simulink model "PassStBkReclnCtrl"  (R2018b)
settings: Solver=FixedStepDiscrete  StartTime=0.0  StopTime=10.0  RelTol=1e-3
undefined symbols (not defined in the file or in its folder): KeSMSuMdMotFinshdTm_Val, KeSMSuMdRetryTm1_Val, KeSMSuModeReqDurgTm_Val
libraries: StCtrlLibBkRecln x1
settings Model: Creator=sn2xws  LastModifiedBy=sn2xws
settings Model: ModifiedHistory=|
  | 2024.6.26 V3.0.0 557模式流程
  | 2024.8.23 V3.0.1更新Entrig接口
  | 2024.11.6 V3.0.2 模式流程V2.6 Md30 增加靠背目标位置1
settings DataIOCC: SaveFormat=StructureWithTime
settings OptimizationCC: DefaultParameterBehavior=Inlined  EnhancedBackFolding=on  PassReuseOutputArgsAs=Individual arguments  ZeroExternalMemoryAtStartup=off  ZeroInternalMemoryAtStartup=off  OptimizeBlockOrder=speed  DifferentSizesBufferReuse=on  OptimizationCustomize=off
settings DebuggingCC: ParameterTunabilityLossMsg=error
settings SFSimCC: MATLABDynamicMemAlloc=off
settings RTWCC: SystemTargetFile=autosar.tlc  GenCodeOnly=on  TemplateMakefile=ert_default_tmf  Description=AUTOSAR  GenerateReport=on  IncludeHyperlinkInReport=on  LaunchReport=on  GenerateTraceInfo=on  GenerateTraceReport=on  GenerateTraceReportSl=on  GenerateTraceReportSf=on  GenerateTraceReportEml=on
settings CodeAppCC: ForceParamTrailComments=on  IgnoreCustomStorageClasses=off  OperatorAnnotations=on  SimulinkDataObjDesc=on  SFDataObjDesc=on  InsertBlockDesc=on
settings STFCustomTargetCC: TargetLangStandard=C99 (ISO)  MultiwordLength=256  ParMdlRefBuildCompliant=on  CompOptLevelCompliant=on  IncludeMdlTerminateFcn=off  CombineOutputUpdateFcns=on  SuppressErrorStatus=on  ERTCustomFileBanners=on  SupportNonFinite=off  SupportComplex=off  SupportContinuousTime=off  SupportNonInlinedSFcns=off  RemoveResetFunc=on  MATLABClassNameForMDSCustomization=Simulink.SoftwareTarget.ERTCustomization  AutosarCompliant=on  UseToolchainInfoCompliant=on  LookupTableObjectStructAxisOrder=2,1,3,4,...  LUTObjectStructOrderEvenSpacing=Size,Table,Breakpoints  SystemTargetFile=autosar.tlc
settings ERTTargetCC: TargetLangStandard=C99 (ISO)  ConcurrentExecutionCompliant=off  IncludeMdlTerminateFcn=off  SuppressErrorStatus=on  SupportNonFinite=off  SupportComplex=off  ModelStepFunctionPrototypeControlCompliant=off  CPPClassGenCompliant=off  AutosarCompliant=on  LookupTableObjectStructAxisOrder=2,1,3,4,...  LUTObjectStructOrderEvenSpacing=Size,Table,Breakpoints  InlinedParameterPlacement=NonHierarchical  ERTCustomFileTemplate=example_file_process.tlc  ERTFilePackagingFormat=Compact

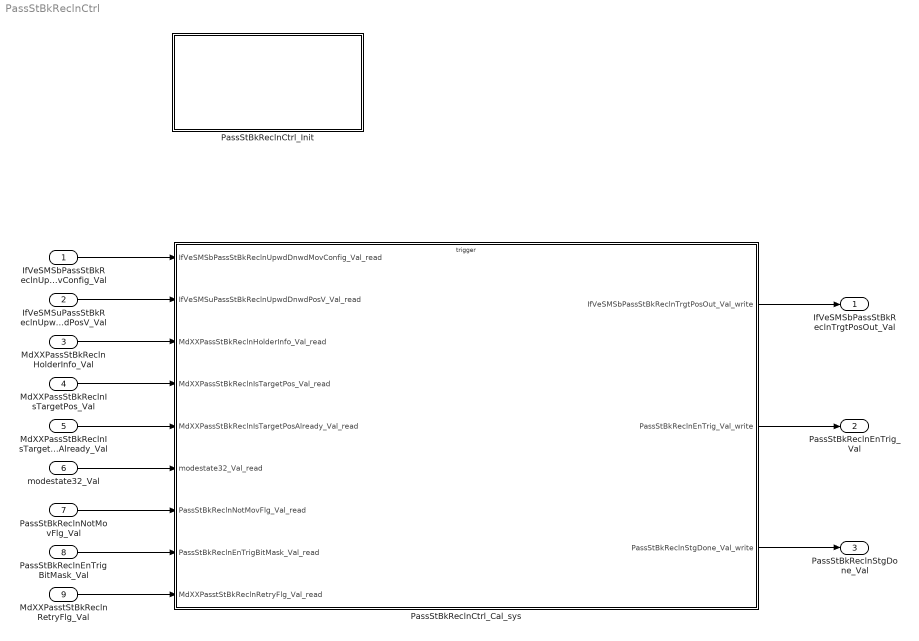
== system PassStBkReclnCtrl ==
  IfVeSMSbPassStBkReclnUpwdDnwdMovConfig_Val : Inport  OutDataTypeStr=boolean  PortDimensions=1
  IfVeSMSuPassStBkReclnUpwdDnwdPosV_Val : Inport  Port=2  OutDataTypeStr=boolean  PortDimensions=1
  MdXXPassStBkReclnHolderInfo_Val : Inport  Port=3  OutDataTypeStr=uint32  PortDimensions=1
  MdXXPassStBkReclnIsTargetPos_Val : Inport  Port=4  OutDataTypeStr=uint32  PortDimensions=1
  MdXXPassStBkReclnIsTargetPosAlready_Val : Inport  Port=5  OutDataTypeStr=uint32  PortDimensions=1
  modestate32_Val : Inport  Port=6  OutDataTypeStr=uint32  PortDimensions=1
  PassStBkReclnNotMovFlg_Val : Inport  Port=7  OutDataTypeStr=boolean  PortDimensions=1
  PassStBkReclnEnTrigBitMask_Val : Inport  Port=8  OutDataTypeStr=uint32  PortDimensions=1
  MdXXPasstStBkReclnRetryFlg_Val : Inport  Port=9  OutDataTypeStr=uint32  PortDimensions=1
  PassStBkReclnCtrl_Cal_sys : Subsystem
  PassStBkReclnCtrl_Init : Subsystem
  IfVeSMSbPassStBkReclnTrgtPosOut_Val : Outport  OutDataTypeStr=boolean  PortDimensions=1
  PassStBkReclnEnTrig_Val : Outport  Port=2  OutDataTypeStr=boolean  PortDimensions=1
  PassStBkReclnStgDone_Val : Outport  Port=3  OutDataTypeStr=boolean  PortDimensions=1
  wires:
  IfVeSMSbPassStBkReclnUpwdDnwdMovConfig_Val/1 -> PassStBkReclnCtrl_Cal_sys/1(IfVeSMSbPassStBkReclnUpwdDnwdMovConfig_Val_read)
  IfVeSMSuPassStBkReclnUpwdDnwdPosV_Val/1 -> PassStBkReclnCtrl_Cal_sys/2(IfVeSMSuPassStBkReclnUpwdDnwdPosV_Val_read)
  MdXXPassStBkReclnHolderInfo_Val/1 -> PassStBkReclnCtrl_Cal_sys/3(MdXXPassStBkReclnHolderInfo_Val_read)
  MdXXPassStBkReclnIsTargetPos_Val/1 -> PassStBkReclnCtrl_Cal_sys/4(MdXXPassStBkReclnIsTargetPos_Val_read)
  MdXXPassStBkReclnIsTargetPosAlready_Val/1 -> PassStBkReclnCtrl_Cal_sys/5(MdXXPassStBkReclnIsTargetPosAlready_Val_read)
  modestate32_Val/1 -> PassStBkReclnCtrl_Cal_sys/6(modestate32_Val_read)
  PassStBkReclnNotMovFlg_Val/1 -> PassStBkReclnCtrl_Cal_sys/7(PassStBkReclnNotMovFlg_Val_read)
  PassStBkReclnCtrl_Cal_sys/1(IfVeSMSbPassStBkReclnTrgtPosOut_Val_write) -> IfVeSMSbPassStBkReclnTrgtPosOut_Val/1
  PassStBkReclnCtrl_Cal_sys/2(PassStBkReclnEnTrig_Val_write) -> PassStBkReclnEnTrig_Val/1
  PassStBkReclnCtrl_Cal_sys/3(PassStBkReclnStgDone_Val_write) -> PassStBkReclnStgDone_Val/1
  PassStBkReclnEnTrigBitMask_Val/1 -> PassStBkReclnCtrl_Cal_sys/8(PassStBkReclnEnTrigBitMask_Val_read)
  MdXXPasstStBkReclnRetryFlg_Val/1 -> PassStBkReclnCtrl_Cal_sys/9(MdXXPasstStBkReclnRetryFlg_Val_read)

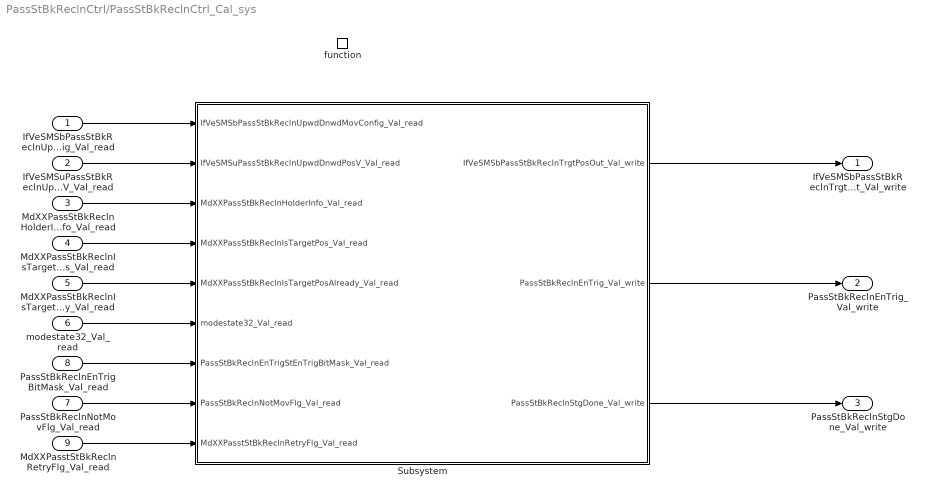
== system PassStBkReclnCtrl/PassStBkReclnCtrl_Cal_sys ==
  IfVeSMSbPassStBkReclnUpwdDnwdMovConfig_Val_read : Inport
  IfVeSMSuPassStBkReclnUpwdDnwdPosV_Val_read : Inport  Port=2
  MdXXPassStBkReclnHolderInfo_Val_read : Inport  Port=3
  MdXXPassStBkReclnIsTargetPos_Val_read : Inport  Port=4
  MdXXPassStBkReclnIsTargetPosAlready_Val_read : Inport  Port=5
  modestate32_Val_read : Inport  Port=6
  PassStBkReclnNotMovFlg_Val_read : Inport  Port=7
  PassStBkReclnEnTrigBitMask_Val_read : Inport  Port=8
  MdXXPasstStBkReclnRetryFlg_Val_read : Inport  Port=9
  function : TriggerPort  TriggerType=function-call  IsSimulinkFunction=on  FunctionName=PassStBkReclnCtrl_Cal  VariantControl=(inherit)
  Subsystem : Subsystem
  IfVeSMSbPassStBkReclnTrgtPosOut_Val_write : Outport
      settings: EnsureOutportIsVirtual=on
  PassStBkReclnEnTrig_Val_write : Outport  Port=2
      settings: EnsureOutportIsVirtual=on
  PassStBkReclnStgDone_Val_write : Outport  Port=3
      settings: EnsureOutportIsVirtual=on
  wires:
  IfVeSMSbPassStBkReclnUpwdDnwdMovConfig_Val_read/1 -> Subsystem/1(IfVeSMSbPassStBkReclnUpwdDnwdMovConfig_Val_read)
  IfVeSMSuPassStBkReclnUpwdDnwdPosV_Val_read/1 -> Subsystem/2(IfVeSMSuPassStBkReclnUpwdDnwdPosV_Val_read)
  MdXXPassStBkReclnHolderInfo_Val_read/1 -> Subsystem/3(MdXXPassStBkReclnHolderInfo_Val_read)
  MdXXPassStBkReclnIsTargetPos_Val_read/1 -> Subsystem/4(MdXXPassStBkReclnIsTargetPos_Val_read)
  MdXXPassStBkReclnIsTargetPosAlready_Val_read/1 -> Subsystem/5(MdXXPassStBkReclnIsTargetPosAlready_Val_read)
  modestate32_Val_read/1 -> Subsystem/6(modestate32_Val_read)
  PassStBkReclnNotMovFlg_Val_read/1 -> Subsystem/8(PassStBkReclnNotMovFlg_Val_read)
  Subsystem/1(IfVeSMSbPassStBkReclnTrgtPosOut_Val_write) -> IfVeSMSbPassStBkReclnTrgtPosOut_Val_write/1
  Subsystem/2(PassStBkReclnEnTrig_Val_write) -> PassStBkReclnEnTrig_Val_write/1
  Subsystem/3(PassStBkReclnStgDone_Val_write) -> PassStBkReclnStgDone_Val_write/1
  PassStBkReclnEnTrigBitMask_Val_read/1 -> Subsystem/7(PassStBkReclnEnTrigStEnTrigBitMask_Val_read)
  MdXXPasstStBkReclnRetryFlg_Val_read/1 -> Subsystem/9(MdXXPasstStBkReclnRetryFlg_Val_read)

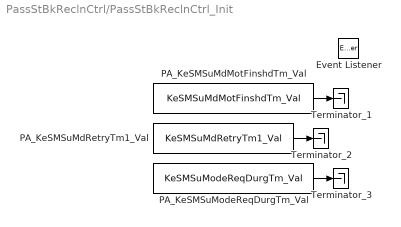
== system PassStBkReclnCtrl/PassStBkReclnCtrl_Init ==
  Event Listener : EventListener  EventName=reset
  PA_KeSMSuMdMotFinshdTm_Val : Constant  Value=KeSMSuMdMotFinshdTm_Val
  PA_KeSMSuMdRetryTm1_Val : Constant  Value=KeSMSuMdRetryTm1_Val
  PA_KeSMSuModeReqDurgTm_Val : Constant  Value=KeSMSuModeReqDurgTm_Val
  Terminator_1 : Terminator
  Terminator_2 : Terminator
  Terminator_3 : Terminator
  wires:
  PA_KeSMSuMdMotFinshdTm_Val/1 -> Terminator_1/1
  PA_KeSMSuMdRetryTm1_Val/1 -> Terminator_2/1
  PA_KeSMSuModeReqDurgTm_Val/1 -> Terminator_3/1

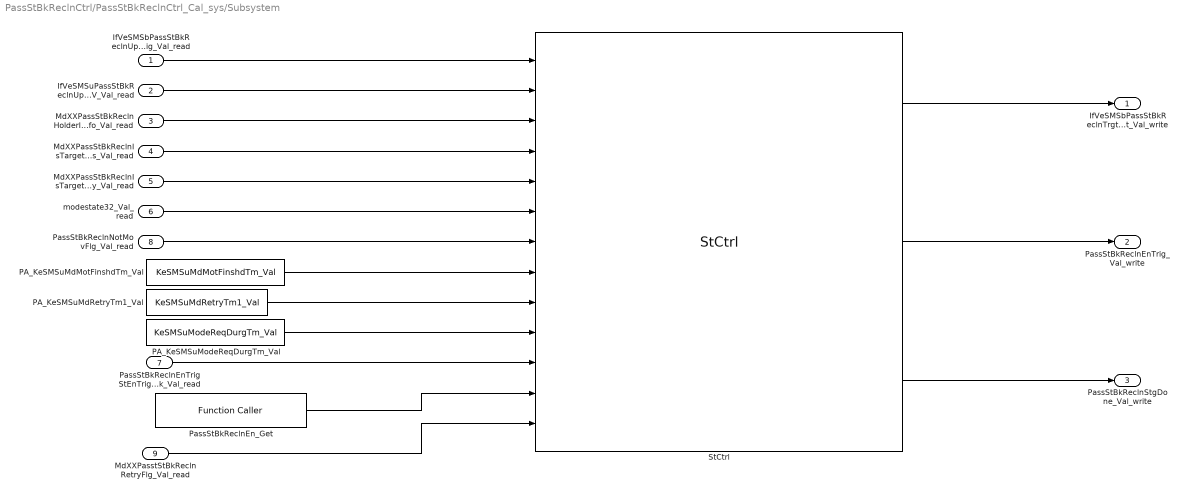
== system PassStBkReclnCtrl/PassStBkReclnCtrl_Cal_sys/Subsystem ==
  IfVeSMSbPassStBkReclnUpwdDnwdMovConfig_Val_read : Inport
  IfVeSMSuPassStBkReclnUpwdDnwdPosV_Val_read : Inport  Port=2
  MdXXPassStBkReclnHolderInfo_Val_read : Inport  Port=3
  MdXXPassStBkReclnIsTargetPos_Val_read : Inport  Port=4
  MdXXPassStBkReclnIsTargetPosAlready_Val_read : Inport  Port=5
  modestate32_Val_read : Inport  Port=6
  PassStBkReclnEnTrigStEnTrigBitMask_Val_read : Inport  Port=7
  PassStBkReclnNotMovFlg_Val_read : Inport  Port=8
  MdXXPasstStBkReclnRetryFlg_Val_read : Inport  Port=9
  PA_KeSMSuMdMotFinshdTm_Val : Constant  Value=KeSMSuMdMotFinshdTm_Val
  PA_KeSMSuMdRetryTm1_Val : Constant  Value=KeSMSuMdRetryTm1_Val
  PA_KeSMSuModeReqDurgTm_Val : Constant  Value=KeSMSuModeReqDurgTm_Val
  PassStBkReclnEn_Get : FunctionCaller  FunctionPrototype=data = PassStBkReclnEn_Get()  OutputArgumentSpecifications=uint32(1)
  StCtrl : StCtrlLibBkRecln/StCtrl  SystemSampleTime=-1
  IfVeSMSbPassStBkReclnTrgtPosOut_Val_write : Outport
      settings: EnsureOutportIsVirtual=on
  PassStBkReclnEnTrig_Val_write : Outport  Port=2
      settings: EnsureOutportIsVirtual=on
  PassStBkReclnStgDone_Val_write : Outport  Port=3
      settings: EnsureOutportIsVirtual=on
  wires:
  PassStBkReclnEn_Get/1 -> StCtrl/12
  StCtrl/1 -> IfVeSMSbPassStBkReclnTrgtPosOut_Val_write/1
  StCtrl/3 -> PassStBkReclnStgDone_Val_write/1
  StCtrl/2 -> PassStBkReclnEnTrig_Val_write/1
  IfVeSMSbPassStBkReclnUpwdDnwdMovConfig_Val_read/1 -> StCtrl/1
  IfVeSMSuPassStBkReclnUpwdDnwdPosV_Val_read/1 -> StCtrl/2
  MdXXPassStBkReclnHolderInfo_Val_read/1 -> StCtrl/3
  MdXXPassStBkReclnIsTargetPos_Val_read/1 -> StCtrl/4
  MdXXPassStBkReclnIsTargetPosAlready_Val_read/1 -> StCtrl/5
  modestate32_Val_read/1 -> StCtrl/6
  PassStBkReclnNotMovFlg_Val_read/1 -> StCtrl/7
  PA_KeSMSuMdMotFinshdTm_Val/1 -> StCtrl/8
  PA_KeSMSuMdRetryTm1_Val/1 -> StCtrl/9
  PA_KeSMSuModeReqDurgTm_Val/1 -> StCtrl/10
  PassStBkReclnEnTrigStEnTrigBitMask_Val_read/1 -> StCtrl/11
  MdXXPasstStBkReclnRetryFlg_Val_read/1 -> StCtrl/13
